simulink model "GNC"  (R2026b)
settings: Solver=VariableStepAuto  StopTime=80  MaxStep=0.01
libraries: simulink x1, slpidlib x1
settings Model: Creator=theog  LastModifiedBy=Jeevan

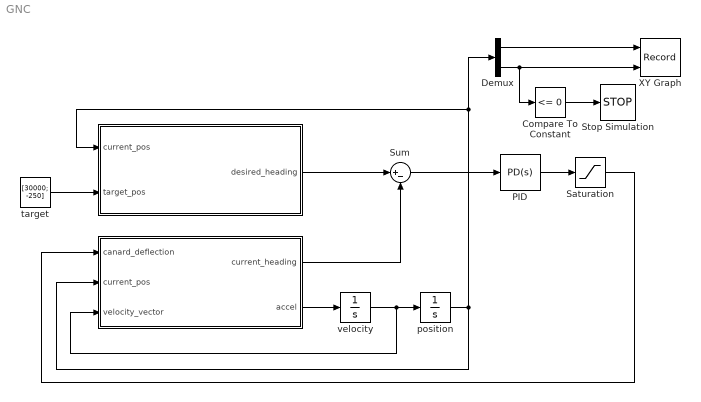
== system GNC ==
  " " : MATLAB Function  TreatAsAtomicUnit=on
  "  " : MATLAB Function  TreatAsAtomicUnit=on
  Compare To Constant : simulink/Logic and Bit Operations/Compare To Constant  relop=<=  const=0  OutDataTypeStr=boolean
  Demux : Demux  Outputs=2
  PID : slpidlib/PID Controller  Controller=PD  Form=Parallel  TimeDomain=Continuous-time  UseExternalTs=off  SampleTime=-1  IntegratorMethod=Forward Euler  FilterMethod=Forward Euler  ControllerParametersSource=internal  P=0.25  I=1  UseKiTs=off  D=0.05  UseExternalDerivativeSource=off  N=100  UseFilter=on  TunerSelectOption=Transfer Function Based (PID Tuner App)  InitialConditionSource=internal  InitialConditionForIntegrator=0  InitialConditionForFilter=0  DifferentiatorICPrevScaledInput=0  ExternalReset=none  TrackingMode=off  Kt=1  LimitOutput=off  SatLimitsSource=internal  UpperSaturationLimit=inf  LowerSaturationLimit=-inf  LinearizeAsGain=on  AntiWindupMode=none  Kb=1  LimitIntegrator=off  UpperIntegratorSaturationLimit=inf  LowerIntegratorSaturationLimit=-inf  POutMin=[]  POutMax=[]  IOutMin=[]  IOutMax=[]  DOutMin=[]  DOutMax=[]  NOutMin=[]  NOutMax=[]  SumOutMin=[]  SumOutMax=[]  SaturationOutMin=[]  SaturationOutMax=[]  PParamMin=[]  PParamMax=[]  IParamMin=[]  IParamMax=[]  DParamMin=[]  DParamMax=[]  NParamMin=[]  NParamMax=[]  KbParamMin=[]  KbParamMax=[]  KtParamMin=[]  KtParamMax=[]  KbOutMin=[]  KbOutMax=[]  KtOutMin=[]  KtOutMax=[]  IntegratorOutMin=[]  IntegratorOutMax=[]  FilterOutMin=[]  FilterOutMax=[]  SumI1OutMin=[]  SumI1OutMax=[]  SumI2OutMin=[]  SumI2OutMax=[]  SumI3OutMin=[]  SumI3OutMax=[]  SumI4OutMin=[]  SumI4OutMax=[]  SumDOutMin=[]  SumDOutMax=[]  DifferentiatorOutMin=[]  DifferentiatorOutMax=[]  FilterDiffOutCoefMin=[]  FilterDiffOutCoefMax=[]  ReciprocalOutMin=[]  ReciprocalOutMax=[]  SumDenOutMin=[]  SumDenOutMax=[]  SumNumOutMin=[]  SumNumOutMax=[]  DivideOutMin=[]  DivideOutMax=[]  UdiffTsProdOutMin=[]  UdiffTsProdOutMax=[]  NTsProdOutMin=[]  NTsProdOutMax=[]  UintegralTsProdOutMin=[]  UintegralTsProdOutMax=[]  UngainTsProdOutMin=[]  UngainTsProdOutMax=[]  ClampingZeroOutDataTypeStr=Inherit: Inherit via back propagation  ClampingZeroOutMin=[]  ClampingZeroOutMax=[]  FilterDenConstantOutDataTypeStr=Inherit: Inherit via back propagation  FilterDenConstantOutMin=[]  FilterDenConstantOutMax=[]  PCopyOutDataTypeStr=Inherit: Inherit via back propagation  PCopyOutMin=[]  PCopyOutMax=[]  NCopyOutDataTypeStr=Inherit: Inherit via back propagation  NCopyOutMin=[]  NCopyOutMax=[]  IntegratorContinuousStateAttributes=''  IntegratorStateMustResolveToSignalObject=off  IntegratorRTWStateStorageClass=Auto  FilterContinuousStateAttributes=''  FilterStateMustResolveToSignalObject=off  FilterRTWStateStorageClass=Auto  ParallelPVariant=InternalParameters  IdealPVariant=Disabled  IVariant=Disabled  DVariant=InternalParameters  IntegratorVariant=Disabled  SatVariant=Disabled  AWVariant=Disabled  PCopyVariant=Disabled  TRVariant=Disabled  FdbkBlocksVariant=Forward  IdealPFdbkVariant=Disabled  SatFdbkVariant=Disabled  DerivativeFilterVariant=ContFilter  NVariant=InternalParameters  NCopyVariant=Disabled  FilterICVariant=InternalICsFilter  IntegratorICVariant=Disabled  ExternalResetVariant=Disabled  TRSumVariant=Passthrough  SumFdbkVariant=Disabled  SumVariant=Sum_PD  TsampFilterVariant=InternalTs  TsampNgainVariant=Passthrough  TsampIntegralVariant=Disabled_SignalSpec  ExternalSaturationOutDataTypeStr=Inherit: Same as second input  DerivativeSourceVariant=ErrorSignal  PreIntVariant=InternalPreInt
  Saturation : Saturate  UpperLimit=0.26  LowerLimit=-0.26
  Stop Simulation : Stop
  Sum : Sum  Inputs=|+-
  XY Graph : Record  NumPorts=2.0  FileSettingsInternal="{\"entries\":[{\"content\":{\"excelSettings\":{\"content\":{},\"type\":\"Streamout.ExcelSettings\"},\"parquetSettings\":{\"content\":{},\"type\":\"Streamout.ParquetSettings\"}},\"type\":\"Streamout.FileSettingStorage\",\"uuid\":\"\"}],\"packageUris\":[\"http:\\/\\/schema.mathworks.com\\/mf0\\/streamout_blocks\\/R2020a\"],\"version\":\"1.0\"}"  FrameSettings=[0, 0]  Layout=[1 1]  SignalsInternal="{\"entries\":[{\"content\":{\"signals\":[{\"content\":{\"blockPath\":[],\"dimensions\":[1],\"domain\":\"\",\"lineColor\":\"#a2142f\",\"plots\":[ 1 ],\"port\":1,\"sid\":[\"\"],\"signalID\":1,\"signalName\":\"Demux:1\"},\"type\":\"RecordBlkView.Signal\",\"uuid\":\"\"},{\"content\":{\"blockPath\":[],\"dimensions\":[1],\"domain\":\"\",\"lineColor\":\"#139fff\",\"plots\":[ 1 ],\"port\":2,\"sid\":[\"\"],\"signalID\":2,\"signalName\":\"Demux:2\"},\"type\":\"RecordBlkView.Signal\",\"uuid\":\"\"}]},\"type\":\"RecordBlkView.InputSignals\",\"uuid\":\"\"}],\"packageUris\":[\"http:\\/\\/schema.mathworks.com\\/mf0\\/streamout_blocks\\/R2020a\"],\"version\":\"1.0\"}"  VisualizationBindings="{\"xyplotplugin\":{\"info\":[{\"series\":[{\"bindingParametersList\":[{\"parameter\":\"X-Axis\",\"signalID\":1,\"signalName\":\"Demux:1\"},{\"parameter\":\"Y-Axis\",\"signalID\":2,\"signalName\":\"Demux:2\"}],\"seriesID\":0},{\"bindingParametersList\":[{\"parameter\":\"X-Axis\",\"signalID\":1,\"signalName\":\"Demux:1\"}],\"seriesID\":1}],\"subplotID\":1}]}}"  CompatibilityTag=XY
  position : Integrator  InitialCondition=[0,1]
  target : Constant  Value=[30000; -250]
  velocity : Integrator  InitialCondition=[655.32; 458.86]
  wires:
  "  "/2(accel) -> velocity/1
  velocity/1 -> position/1, "  "/3(velocity_vector)
  target/1 -> " "/2(target_pos)
  position/1 -> "  "/2(current_pos), " "/1(current_pos), Demux/1
  " "/1(desired_heading) -> Sum/1
  "  "/1(current_heading) -> Sum/2
  Sum/1 -> PID/1
  Demux/1 -> XY Graph/1
  PID/1 -> Saturation/1
  Demux/2 -> XY Graph/2, Compare To Constant/1
  Compare To Constant/1 -> Stop Simulation/1
  Saturation/1 -> "  "/1(canard_deflection)

== matlab function GNC/   ==
  data: current_heading output; accel output; canard_deflection input; current_pos input; velocity_vector input
function [current_heading, accel] = dynamics(canard_deflection, current_pos, velocity_vector)
% 1. Parse current states
vx = velocity_vector(1);
vy = velocity_vector(2);
altitude = max(0, current_pos(2)); % Prevent negative altitude math errors

% 2. REAL-WORLD ATMOSPHERE (ISA MODEL)
% Valid for the Troposphere (up to ~11,000 meters / 36,000 ft)
T0 = 288.15;       % Sea level standard temperature (K)
P0 = 101325;       % Sea level standard pressure (Pa)
L = 0.0065;        % Temperature lapse rate (K/m)
R = 287.05;        % Specific gas constant for air
g = 9.81;          % Gravity

T = T0 - L * altitude;
P = P0 * (T / T0)^(g / (L * R));
rho = P / (R * T); % Dynamic Air Density (kg/m^3)

% 3. WIND & RELATIVE AIRSPEED
% Simulating a constant 15 m/s (54 km/h) horizontal headwind
w_x = -15; 
w_y = 0;

% Aerodynamic forces rely on airspeed, kinematics rely on groundspeed
v_air_x = vx - w_x;
v_air_y = vy - w_y;
v_air_mag = sqrt(v_air_x^2 + v_air_y^2);

% Calculate headings
air_heading = atan2(v_air_y, v_air_x);
current_heading = atan2(vy, vx); 

% 4. DYNAMIC MACH NUMBER & DRAG
gamma = 1.4;
speed_of_sound = sqrt(gamma * R * T);
mach = v_air_mag / speed_of_sound;

% Basic Mach-dependent drag step (Higher drag when supersonic)
if mach > 1.0
    c_d = 0.000004; 
else
    c_d = 0.000002; 
end
k_L = 0.02; 

% Lock fins flat for the first 18km to punch through the lower atmosphere.
if current_pos(1) < 18000
    canard_deflection = 0; 
end

% 5. FORCES & KINEMATICS
% Incorporating dynamic air density (rho) into the force equations
a_drag = c_d * rho * v_air_mag^2;
a_lift = k_L * rho * v_air_mag^2 * canard_deflection;

% Convert aerodynamic forces back into global X and Y accelerations
ax = -a_drag * cos(air_heading) - a_lift * sin(air_heading);
ay = -a_drag * sin(air_heading) + a_lift * cos(air_heading) - g;

accel = [ax; ay];
end

== matlab function GNC/  ==
  data: current_pos input; desired_heading output; target_pos input
function desired_heading = guidance(current_pos, target_pos)
dx = target_pos(1) - current_pos(1);
dy = target_pos(2) - current_pos(2);
desired_heading = atan2(dy, dx);
end
